simulink model "estimacionParametros"  (R2021a)
settings: Solver=ode45  StartTime=0.0  StopTime=10  RelTol=1e-3
values from neighbouring files (symbols this model uses):
  AL = double(subs(A,{R,L,Kv,Ki,n,Jm,Jl,Bm,Bl,m,d,g,x1,x2,x3,Vin},{R0,L0,Kv0,Ki0,n0,Jm0,Jl0,Bm0,Bl0,m0,d0,g0,x10,x20,x30,Vin0}))    [modeloMATEMATICOFINAL.m]
  BL = double(subs(B,{R,L,Kv,Ki,n,Jm,Jl,Bm,Bl,m,d,g,x1,x2,x3,Vin},{R0,L0,Kv0,Ki0,n0,Jm0,Jl0,Bm0,Bl0,m0,d0,g0,x10,x20,x30,Vin0}))    [modeloMATEMATICOFINAL.m]
  CL = [0 1 0 ... (first row only)    [modeloMATEMATICOFINAL.m]
  DL = [0 ... (first row only)    [modeloMATEMATICOFINAL.m]
undefined symbols (not defined in the file or in its folder): Blo, Bmo, do, go, Jlo, Jmo, Kio, Kvo, Lo, mo, no, Ro, X10, X20, X30
settings Model: OrderedModelArguments=off  Creator=hubertdelgado  LastModifiedBy=hubertdelgado

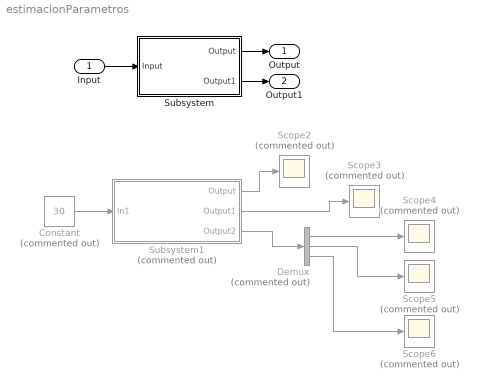
== system estimacionParametros ==
  Input : Inport
  Constant : Constant  Commented=on  Value=30
  Demux : Demux  Commented=on  Outputs=3
  Scope{2..6} (5 alike) : Scope  Commented=on
  Subsystem : Subsystem
  Subsystem1 : Subsystem  Commented=on
  Output : Outport
  Output1 : Outport  Port=2
  wires:
  Demux/1 -> Scope4/1
  Demux/2 -> Scope5/1
  Subsystem1/3(Output2) -> Demux/1
  Demux/3 -> Scope6/1
  Subsystem1/2(Output1) -> Scope3/1
  Subsystem1/1(Output) -> Scope2/1
  Constant/1 -> Subsystem1/1(In1)
  Input/1 -> Subsystem/1(Input)
  Subsystem/1(Output) -> Output/1
  Subsystem/2(Output1) -> Output1/1

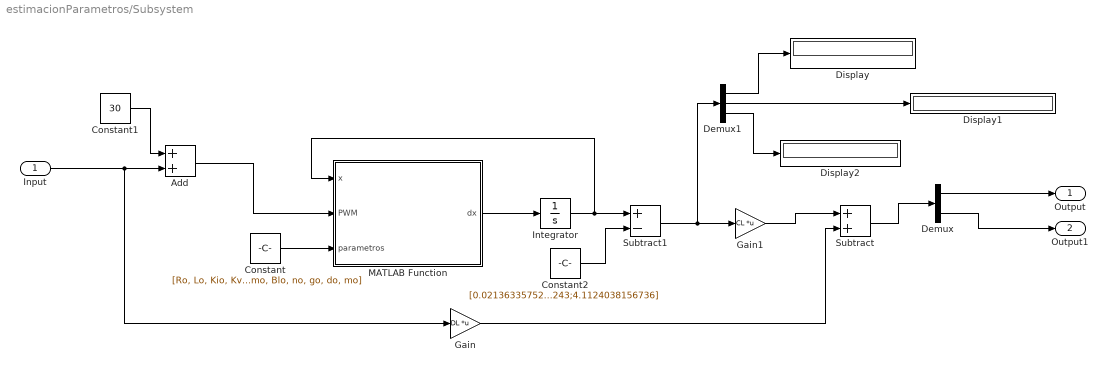
== system estimacionParametros/Subsystem ==
  Input : Inport
  Add : Sum
  Constant : Constant  Value=[Ro, Lo, Kio, Kvo, Jmo, Jlo, Bmo, Blo, no, go, do, mo]
  Constant1 : Constant  Value=30
  Constant2 : Constant  Value=[0.021363357520018;38.80690895243;4.1124038156736]
  Demux : Demux  Outputs=2
  Demux1 : Demux  Outputs=3
  Display : Display
  Display1 : Display
  Display2 : Display
  Gain : Gain  Gain=DL  Multiplication=Matrix(K*u)
  Gain1 : Gain  Gain=CL  Multiplication=Matrix(K*u)
  Integrator : Integrator  InitialCondition=[X10; X20; X30]
  MATLAB Function : MATLAB Function  TreatAsAtomicUnit=on
  Subtract : Sum
  Subtract1 : Sum  Inputs=+-
  Output : Outport
  Output1 : Outport  Port=2
  wires:
  Subtract/1 -> Demux/1
  Gain1/1 -> Subtract/1
  Demux/2 -> Output1/1
  Subtract1/1 -> Demux1/1, Gain1/1
  Integrator/1 -> Subtract1/1, MATLAB Function/1(x)
  Constant/1 -> MATLAB Function/3(parametros)
  MATLAB Function/1(dx) -> Integrator/1
  Demux/1 -> Output/1
  Constant1/1 -> Add/1
  Gain/1 -> Subtract/2
  Constant2/1 -> Subtract1/2
  Add/1 -> MATLAB Function/2(PWM)
  Input/1 -> Gain/1, Add/2
  Demux1/1 -> Display/1
  Demux1/2 -> Display1/1
  Demux1/3 -> Display2/1

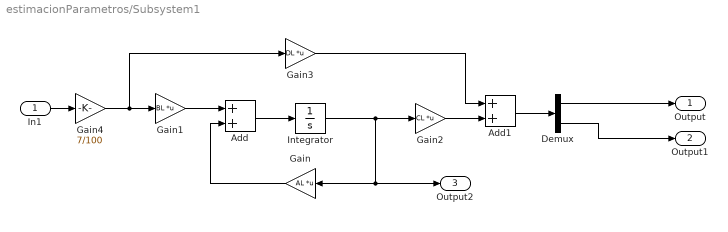
== system estimacionParametros/Subsystem1 ==
  In1 : Inport
  Add : Sum
  Add1 : Sum
  Demux : Demux  Outputs=2
  Gain : Gain  Gain=AL  Multiplication=Matrix(K*u)
  Gain1 : Gain  Gain=BL  Multiplication=Matrix(K*u)
  Gain2 : Gain  Gain=CL  Multiplication=Matrix(K*u)
  Gain3 : Gain  Gain=DL  Multiplication=Matrix(K*u)
  Gain4 : Gain  Gain=7/100
  Integrator : Integrator
  Output : Outport
  Output1 : Outport  Port=2
  Output2 : Outport  Port=3
  wires:
  Integrator/1 -> Gain2/1, Output2/1, Gain/1
  Gain3/1 -> Add1/1
  Add/1 -> Integrator/1
  Gain1/1 -> Add/1
  Add1/1 -> Demux/1
  Gain/1 -> Add/2
  Gain2/1 -> Add1/2
  Demux/2 -> Output1/1
  Demux/1 -> Output/1
  In1/1 -> Gain4/1
  Gain4/1 -> Gain3/1, Gain1/1

== matlab function estimacionParametros/Subsystem/MATLAB Function ==
  data: x input; PWM input; dx output; parametros input
function dx = fcn(x,PWM,parametros)

%ESTADOS
x1 = x(1);
x2 = x(2);
x3 = x(3);

%Parametros
R = parametros(1);
L = parametros(2);
Ki = parametros(3);
Kv = parametros(4);
Jm = parametros(5);
Jl = parametros(6);
Bm = parametros(7);
Bl = parametros(8);
n = parametros(9);
g = parametros(10);
d = parametros(11);
m = parametros(12);

%EXPRESIONES
% Jt = Jm*n^2 +Jl;
% f1 = (1/L)*(((7*PWM)/100) - R*x1 - Kv*x2*n);
% f2 = (1/Jt)*(Ki*x1*n - (Bm*n^2 + Bl)*x2 - m*g*d*sin(x3));
% f3 = x2;

% MODELO 2 ESTADOS I TL WL  SALIDA TL WL
f1 = (((7*PWM)/100)-Kv*x3*n-R*x1)/(L); %di/dt
f2 = x3; %d0l/dt = Wl
f3 = ((Ki*x1*n)-x3*(Bm*n^2+Bl)-(m*g*d*sin(x2)))/(Jl+Jm*n^2);  %dwl/dt 

dx = [f1; f2; f3];
